simulink model "lqr_controller_simulation_for_rocket_landing"  (R2021b)
settings: Solver=VariableStepAuto  StartTime=0.0  StopTime=simulation_time  RelTol=1e-3
values from neighbouring files (symbols this model uses):
  A = [0 1 0 0 0 0 ... (first row only)    [LQR_control.m]
  B = [0 0 ... (first row only)    [LQR_control.m]
  x0 = [1000 ... (first row only)    [LQR_control.m]
undefined symbols (not defined in the file or in its folder): K
settings Model: Creator=atauz  LastModifiedBy=atauz

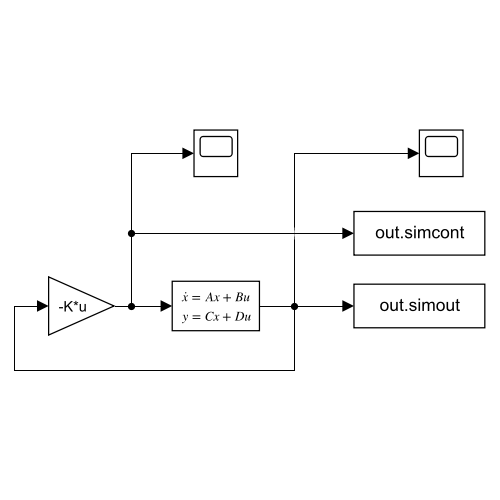
[thumbnail: Simulink's stored preview of the top-level diagram]
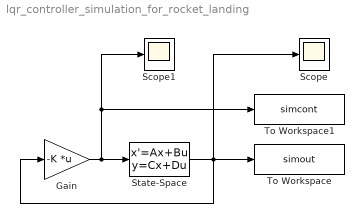
== system lqr_controller_simulation_for_rocket_landing ==
  Gain : Gain  Gain=-K  Multiplication=Matrix(K*u)
  Scope : Scope
  Scope1 : Scope
  State-Space : StateSpace  A=A  B=B  C=eye(6)  D=zeros(6 ,2)  InitialCondition=x0  ParameterTunability=Unconstrained
  To Workspace : ToWorkspace  VariableName=simout  SaveFormat=Structure With Time  SampleTime=-1
  To Workspace1 : ToWorkspace  VariableName=simcont  SaveFormat=Structure With Time  SampleTime=-1
  wires:
  Gain/1 -> Scope1/1, To Workspace1/1, State-Space/1
  State-Space/1 -> To Workspace/1, Gain/1, Scope/1
